simulink model "Control_Validation"  (R2020b)
settings: Solver=VariableStepAuto  StartTime=0.0  StopTime=12  RelTol=1e-3
values from neighbouring files (symbols this model uses):
  A = [5.11995503588 1 0 0 0 0 -11.4260465467 0 1 0 0 0 ... (36 elements, 6x6)]    [Estimated_Model.mat]
  B = [1 0 0 0 0 0]    [Estimated_Model.mat]
  C = [-6.48338492424e-05 0.00041393325507 -0.000527701144131 0.00055117489166 -0.000426728644373 0]    [Estimated_Model.mat]
  D = 0    [Estimated_Model.mat]
  Ts = 1/fs    (= 0.01)    [BasicSim.m]    (also in IdentificationAlgorithm_best.m; LQE_LQR_par.m; demo.m)
undefined symbols (not defined in the file or in its folder): K, M, sigbuilder_block
settings Model: Creator=renato  LastModifiedBy=renato

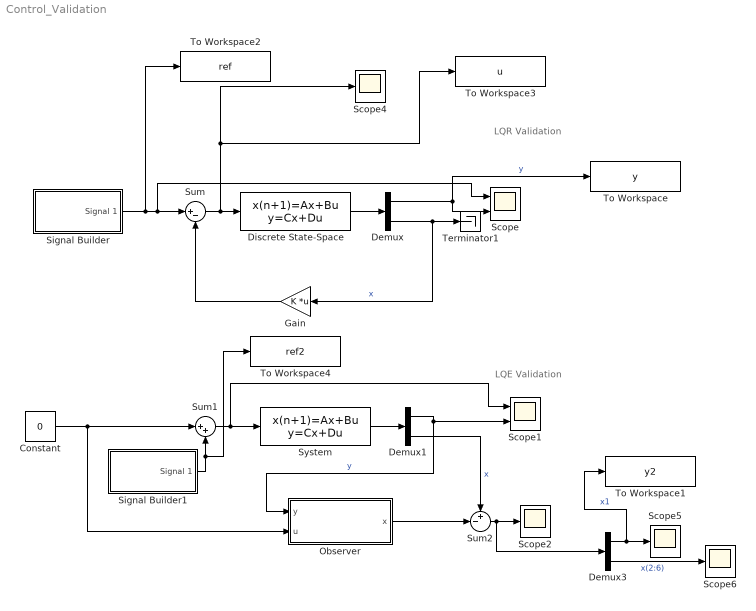
== system Control_Validation ==
  note: LQR Validation
  note: LQE Validation
  Constant : Constant  Value=0
  Demux : Demux  Outputs=[1,6]
  Demux1 : Demux  Outputs=[1,6]
  Demux3 : Demux  Outputs=[1,5]
  Discrete State-Space : DiscreteStateSpace  A=A  B=B  C=[C ; eye(6)]  D=[D; 0;0;0;0;0;0]  SampleTime=0.01
  Gain : Gain  Gain=K  Multiplication=Matrix(K*u)
  Observer : Subsystem
  Scope : Scope  NumInputPorts=2
  Scope1 : Scope  NumInputPorts=2
  Scope{2,4..6} (4 alike) : Scope
  Signal Builder : Subsystem  Tag=STV Subsys  LoadFcn=sigbuilder_block('load');  StartFcn=sigbuilder_block('start');  StopFcn=sigbuilder_block('stop');  ClipboardFcn=sigbuilder_block('clipboard');  mask(Sigbuilder block){tuvar=[0:10]}
      mask help: Simulink:masks:SigbuilderBlock_MD
      mask init:
      | if ~strcmp(get_param(bdroot(gcbh),'SimulationStatus'),'stopped') tuvar = sigbuilder_block('maskInit'); end
      settings: CopyFcn=sigbuilder_block('copy');  DeleteFcn=sigbuilder_block('delete');  ModelCloseFcn=sigbuilder_block('modelClose');  PreSaveFcn=sigbuilder_block('preSave');  PauseFcn=sigbuilder_block('pause');  ContinueFcn=sigbuilder_block('continue');  NameChangeFcn=sigbuilder_block('namechange');  OpenFcn=sigbuilder_block('open',[612.75 227.25 558 354.75 ]);  CloseFcn=sigbuilder_block('close');
      mask Display: plot(0, 0, 100, 100,[2, 2, 32, 32, 2], [68, 8, 8, 68, 68],[32, 2], [38, 38], [32, 19, 2],[53, 60, 44], [32, 17, 17, 2],[16, 16, 31, 31]);txt = getActiveGroup(gcbh);text(2, 100, txt,'verticalAlignment', 'top');
  Signal Builder1 : Subsystem  Tag=STV Subsys  LoadFcn=sigbuilder_block('load');  StartFcn=sigbuilder_block('start');  StopFcn=sigbuilder_block('stop');  ClipboardFcn=sigbuilder_block('clipboard');  mask(Sigbuilder block){tuvar=[0:10]}
      mask help: Simulink:masks:SigbuilderBlock_MD
      mask init:
      | if ~strcmp(get_param(bdroot(gcbh),'SimulationStatus'),'stopped') tuvar = sigbuilder_block('maskInit'); end
      settings: CopyFcn=sigbuilder_block('copy');  DeleteFcn=sigbuilder_block('delete');  ModelCloseFcn=sigbuilder_block('modelClose');  PreSaveFcn=sigbuilder_block('preSave');  PauseFcn=sigbuilder_block('pause');  ContinueFcn=sigbuilder_block('continue');  NameChangeFcn=sigbuilder_block('namechange');  OpenFcn=sigbuilder_block('open',[590.25 177 558 354.75 ]);  CloseFcn=sigbuilder_block('close');
      mask Display: plot(0, 0, 100, 100,[2, 2, 32, 32, 2], [68, 8, 8, 68, 68],[32, 2], [38, 38], [32, 19, 2],[53, 60, 44], [32, 17, 17, 2],[16, 16, 31, 31]);txt = getActiveGroup(gcbh);text(2, 100, txt,'verticalAlignment', 'top');
  Sum : Sum  Inputs=|+-
  Sum1 : Sum  Inputs=|++
  Sum2 : Sum  Inputs=+-|
  System : DiscreteStateSpace  A=A  B=B  C=[C ; eye(6)]  D=[D; 0;0;0;0;0;0]  SampleTime=0.01
  Terminator1 : Terminator
  To Workspace : ToWorkspace  VariableName=y  SaveFormat=Timeseries  SampleTime=-1
  To Workspace1 : ToWorkspace  VariableName=y2  SaveFormat=Timeseries  SampleTime=-1
  To Workspace2 : ToWorkspace  VariableName=ref  SaveFormat=Timeseries  SampleTime=-1
  To Workspace3 : ToWorkspace  VariableName=u  SaveFormat=Timeseries  SampleTime=-1
  To Workspace4 : ToWorkspace  VariableName=ref2  SaveFormat=Timeseries  SampleTime=-1
  wires:
  Discrete State-Space/1 -> Demux/1
  Demux/1 -> To Workspace/1, Scope/2  "y"
  Demux/2 -> Gain/1, Terminator1/1  "x"
  Signal Builder/1(Signal 1) -> To Workspace2/1, Scope/1, Sum/1
  Sum/1 -> To Workspace3/1, Scope4/1, Discrete State-Space/1
  Gain/1 -> Sum/2
  Demux1/1 -> Observer/1(y), Scope1/2  "y"
  System/1 -> Demux1/1
  Demux1/2 -> Sum2/1  "x"
  Signal Builder1/1(Signal 1) -> To Workspace4/1, Sum1/2
  Sum1/1 -> Scope1/1, System/1
  Constant/1 -> Observer/2(u), Sum1/1
  Observer/1(x) -> Sum2/2
  Sum2/1 -> Demux3/1, Scope2/1
  Demux3/1 -> To Workspace1/1, Scope5/1  "x1"
  Demux3/2 -> Scope6/1  "x(2:6)"

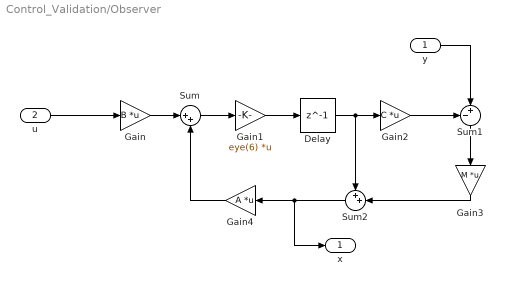
== system Control_Validation/Observer ==
  y : Inport
  u : Inport  Port=2
  Delay : Delay  DelayLength=1  SampleTime=Ts
  Gain : Gain  Gain=B  Multiplication=Matrix(K*u)
  Gain1 : Gain  Gain=eye(6)  Multiplication=Matrix(K*u)
  Gain2 : Gain  Gain=C  Multiplication=Matrix(K*u)
  Gain3 : Gain  Gain=M  Multiplication=Matrix(K*u)
  Gain4 : Gain  Gain=A  Multiplication=Matrix(K*u)
  Sum : Sum  Inputs=|++
  Sum1 : Sum  Inputs=-+|
  Sum2 : Sum  Inputs=++|
  x : Outport
  wires:
  u/1 -> Gain/1
  Gain/1 -> Sum/1
  Sum/1 -> Gain1/1
  Gain1/1 -> Delay/1
  Delay/1 -> Sum2/1, Gain2/1
  Gain2/1 -> Sum1/1
  y/1 -> Sum1/2
  Sum1/1 -> Gain3/1
  Gain4/1 -> Sum/2
  Sum2/1 -> x/1, Gain4/1
  Gain3/1 -> Sum2/2

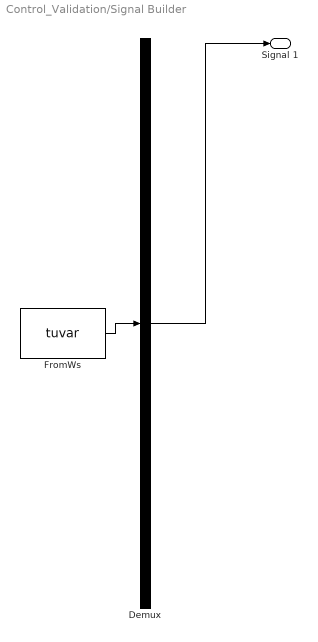
== system Control_Validation/Signal Builder ==
  Demux : Demux  Tag=STV Demux  Outputs=1
      settings: DisplayOption=none
  FromWs : FromWorkspace  Tag=STV FromWs  VariableName=tuvar
      SigBuilderData=|
      | common.afterFinalStr = 'Extrapolate'
      | common.sampleTime = 0
      | dataSet.timeRange = [0 20]
      | dataSet.name = 'Group 1'
      | sbobj.Groups.Name = 'Group 1'
      | sbobj.Groups.Signals.Name = 'Signal 1'
      | sbobj.Groups.Signals.XData = [0 1 1 14.05 14.05 20]
      | sbobj.Groups.Signals.YData = [0 0 1 1 0 0]
      | sbobj.Groups.TimeRange = [0 20]
  Signal 1 : Outport  Tag=STV Outport
  wires:
  Demux/1 -> Signal 1/1
  FromWs/1 -> Demux/1

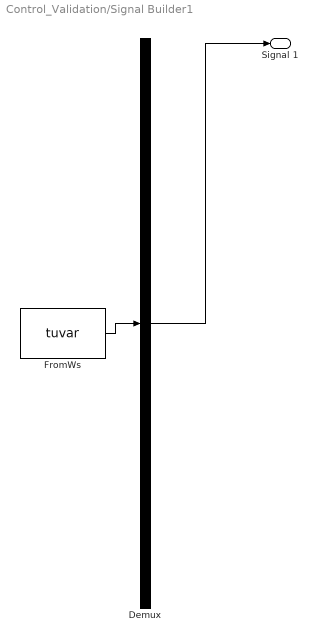
== system Control_Validation/Signal Builder1 ==
  Demux : Demux  Tag=STV Demux  Outputs=1
      settings: DisplayOption=none
  FromWs : FromWorkspace  Tag=STV FromWs  VariableName=tuvar
      SigBuilderData=|
      | common.afterFinalStr = 'Extrapolate'
      | common.sampleTime = 0
      | dataSet.timeRange = [0 10]
      | dataSet.name = 'Group 1'
      | sbobj.Groups.Name = 'Group 1'
      | sbobj.Groups.Signals.Name = 'Signal 1'
      | sbobj.Groups.Signals.XData = [0 1 1 7 7 10]
      | sbobj.Groups.Signals.YData = [0 0 1 1 0 0]
  Signal 1 : Outport  Tag=STV Outport
  wires:
  Demux/1 -> Signal 1/1
  FromWs/1 -> Demux/1
